simulink model "PowertrainElectrical"  (R2025a)
settings: Solver=VariableStepAuto  StartTime=0.0  StopTime=60  RelTol=1e-3
undefined symbols (not defined in the file): canChannel, Data, ID, Ts_PID, w_max
libraries: canlib x3, ESys x3, simulink x1, slpidlib x1
settings Model: DataDictionary=System.sldd  Creator=tecnicomcbti  LastModifiedBy=tecnicomcbti

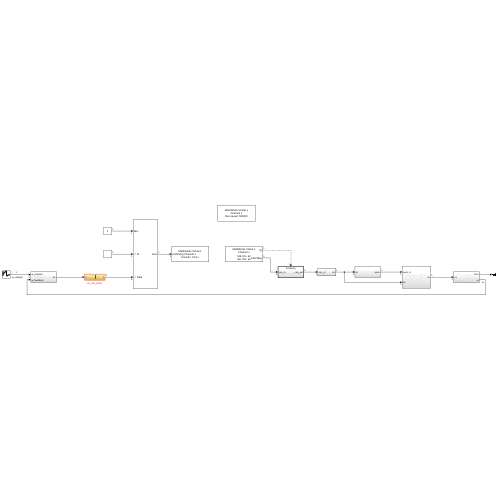
[thumbnail: Simulink's stored preview of the top-level diagram]
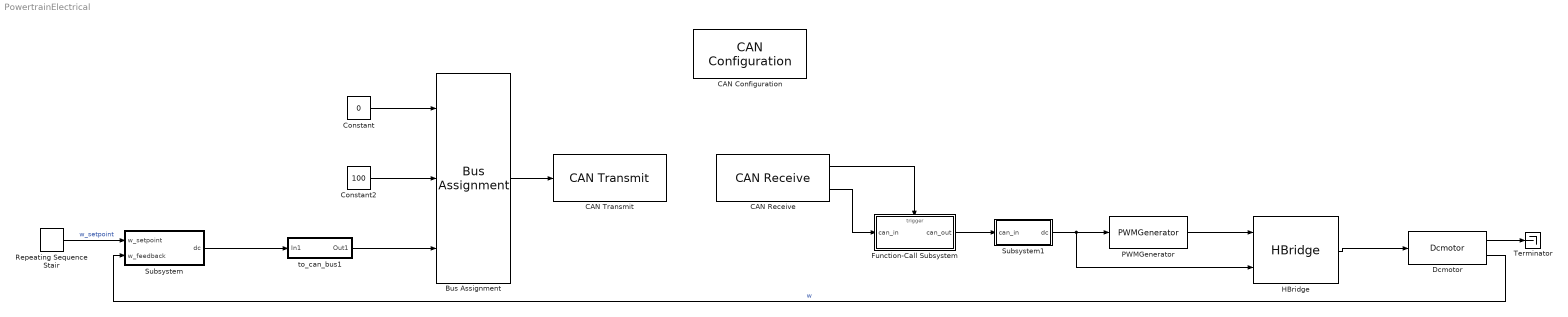
== system PowertrainElectrical ==
  Bus Assignment : BusAssignment  AssignedSignals=ID,Data
  CAN Configuration : canlib/CAN Configuration  BlockHandle=224.0002  Device=MathWorks Virtual 1 (Channel 1)  DeviceMenu=MathWorks Virtual 1 (Channel 1)  ObjConstructor=canChannel('MathWorks', 'Virtual 1', 1)  BusSpeed=500000  EnableBitParameters=off  AckMode=Normal
  CAN Receive : canlib/CAN Receive  BlockHandle=225.0002  Device=MathWorks Virtual 1 (Channel 1)  DeviceMenu=MathWorks Virtual 1 (Channel 1)  ObjConstructor=canChannel('MathWorks', 'Virtual 1', 1)  EnableStandardIDsFilter=off  StdIDsCombo=Allow all  StandardIDs=0  EnableExtendedIDsFilter=off  ExtIDsCombo=Allow all  ExtendedIDs=0  SampleTime=10e-3  MsgsPerTimestep=1  InternalFilterUpdateStatus=on  BusOutput=on
  CAN Transmit : canlib/CAN Transmit  BlockHandle=228.0001  Device=MathWorks Virtual 1 (Channel 1)  DeviceMenu=MathWorks Virtual 1 (Channel 1)  ObjConstructor=canChannel('MathWorks', 'Virtual 1', 1)  EnableEventTransmit=off  EnablePeriodicTransmit=on  MessagePeriod=10e-3
  Constant : Constant  Value=0  OutDataTypeStr=Bus: CAN_MESSAGE_BUS
  Constant2 : Constant  Value=100  OutDataTypeStr=uint32
  Dcmotor : ESys/Dcmotor  SystemSampleTime=-1  VariantActivationTime=update diagram  EmptyChoice=off  PassThrough=off  PassThroughVariantControl=(default)  EmptyChoiceVariantControl=(default)  AllowFlexibleInterface=on  Latency=0  AutoFrameSizeCalculation=off
  Function-Call Subsystem : Subsystem  TreatAsAtomicUnit=on
  HBridge : ESys/HBridge  SystemSampleTime=-1  VariantActivationTime=update diagram  EmptyChoice=off  PassThrough=off  PassThroughVariantControl=(default)  EmptyChoiceVariantControl=(default)  AllowFlexibleInterface=on  Latency=0  AutoFrameSizeCalculation=off
  PWMGenerator : ESys/PWMGenerator  SystemSampleTime=-1  VariantActivationTime=update diagram  EmptyChoice=off  PassThrough=off  PassThroughVariantControl=(default)  EmptyChoiceVariantControl=(default)  AllowFlexibleInterface=on  Latency=0  AutoFrameSizeCalculation=off
  Repeating Sequence Stair : simulink/Sources/Repeating Sequence Stair  OutValues=[300 400 500 150 200 250].'  tsamp=10  OutMin=[]  OutMax=[]  OutDataTypeStr=double  OutputDataTypeScalingMode=double  OutDataType=fixdt(0,8)  ConRadixGroup=Best Precision: Vector-wise  OutScaling=2^-12
  Subsystem : Subsystem
  Subsystem1 : Subsystem
  Terminator : Terminator
  to_can_bus1 : Subsystem
  wires:
  CAN Receive/2 -> Function-Call Subsystem/1(can_in)
  Function-Call Subsystem/1(can_out) -> Subsystem1/1(can_in)
  Bus Assignment/1 -> CAN Transmit/1
  Constant2/1 -> Bus Assignment/2
  CAN Receive/1 -> Function-Call Subsystem/Trigger
  Repeating Sequence Stair/1 -> Subsystem/1(w_setpoint)  "w_setpoint"
  Subsystem/1(dc) -> to_can_bus1/1(In1)
  Subsystem1/1(dc) -> HBridge/2, PWMGenerator/1
  PWMGenerator/1 -> HBridge/1
  HBridge/1 -> Dcmotor/1
  Dcmotor/2 -> Subsystem/2(w_feedback)  "w"
  Dcmotor/1 -> Terminator/1
  Constant/1 -> Bus Assignment/1
  to_can_bus1/1(Out1) -> Bus Assignment/3

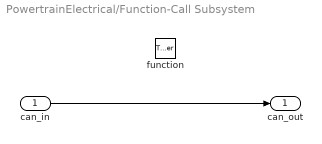
== system PowertrainElectrical/Function-Call Subsystem ==
  can_in : Inport
  function : TriggerPort  TriggerType=function-call  VariantControl=(inherit)
  can_out : Outport
  wires:
  can_in/1 -> can_out/1

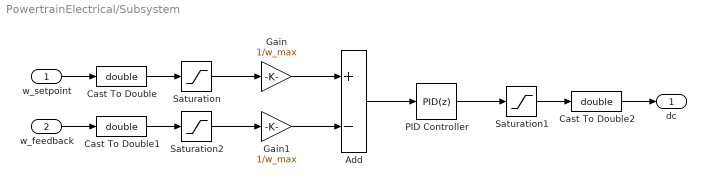
== system PowertrainElectrical/Subsystem ==
  w_setpoint : Inport
  w_feedback : Inport  Port=2
  Add : Sum  Inputs=+-
  Cast To Double : DataTypeConversion  OutDataTypeStr=double  SaturateOnIntegerOverflow=off  RndMeth=Floor
  Cast To Double1 : DataTypeConversion  OutDataTypeStr=double  SaturateOnIntegerOverflow=off  RndMeth=Floor
  Cast To Double2 : DataTypeConversion  OutDataTypeStr=double  SaturateOnIntegerOverflow=off  RndMeth=Floor
  Gain : Gain  Gain=1/w_max
  Gain1 : Gain  Gain=1/w_max
  PID Controller : slpidlib/PID Controller  Controller=PID  Form=Parallel  TimeDomain=Discrete-time  UseExternalTs=off  SampleTime=Ts_PID  IntegratorMethod=Forward Euler  FilterMethod=Forward Euler  ControllerParametersSource=internal  P=0.00488937991617763  I=0.977875983235526  UseKiTs=off  D=0  UseExternalDerivativeSource=off  N=100  UseFilter=on  TunerSelectOption=Transfer Function Based (PID Tuner App)  InitialConditionSource=internal  InitialConditionForIntegrator=0  InitialConditionForFilter=0  DifferentiatorICPrevScaledInput=0  ExternalReset=none  TrackingMode=off  Kt=1  LimitOutput=off  SatLimitsSource=internal  UpperSaturationLimit=inf  LowerSaturationLimit=-inf  LinearizeAsGain=on  AntiWindupMode=none  Kb=1  LimitIntegrator=off  UpperIntegratorSaturationLimit=inf  LowerIntegratorSaturationLimit=-inf  POutMin=[]  POutMax=[]  IOutMin=[]  IOutMax=[]  DOutMin=[]  DOutMax=[]  NOutMin=[]  NOutMax=[]  SumOutMin=[]  SumOutMax=[]  SaturationOutMin=[]  SaturationOutMax=[]  PParamMin=[]  PParamMax=[]  IParamMin=[]  IParamMax=[]  DParamMin=[]  DParamMax=[]  NParamMin=[]  NParamMax=[]  KbParamMin=[]  KbParamMax=[]  KtParamMin=[]  KtParamMax=[]  KbOutMin=[]  KbOutMax=[]  KtOutMin=[]  KtOutMax=[]  IntegratorOutMin=[]  IntegratorOutMax=[]  FilterOutMin=[]  FilterOutMax=[]  SumI1OutMin=[]  SumI1OutMax=[]  SumI2OutMin=[]  SumI2OutMax=[]  SumI3OutMin=[]  SumI3OutMax=[]  SumI4OutMin=[]  SumI4OutMax=[]  SumDOutMin=[]  SumDOutMax=[]  DifferentiatorOutMin=[]  DifferentiatorOutMax=[]  FilterDiffOutCoefMin=[]  FilterDiffOutCoefMax=[]  ReciprocalOutMin=[]  ReciprocalOutMax=[]  SumDenOutMin=[]  SumDenOutMax=[]  SumNumOutMin=[]  SumNumOutMax=[]  DivideOutMin=[]  DivideOutMax=[]  UdiffTsProdOutMin=[]  UdiffTsProdOutMax=[]  NTsProdOutMin=[]  NTsProdOutMax=[]  UintegralTsProdOutMin=[]  UintegralTsProdOutMax=[]  UngainTsProdOutMin=[]  UngainTsProdOutMax=[]  ClampingZeroOutDataTypeStr=Inherit: Inherit via back propagation  ClampingZeroOutMin=[]  ClampingZeroOutMax=[]  FilterDenConstantOutDataTypeStr=Inherit: Inherit via back propagation  FilterDenConstantOutMin=[]  FilterDenConstantOutMax=[]  PCopyOutDataTypeStr=Inherit: Inherit via back propagation  PCopyOutMin=[]  PCopyOutMax=[]  NCopyOutDataTypeStr=Inherit: Inherit via back propagation  NCopyOutMin=[]  NCopyOutMax=[]  IntegratorContinuousStateAttributes=''  IntegratorStateMustResolveToSignalObject=off  IntegratorRTWStateStorageClass=Auto  FilterContinuousStateAttributes=''  FilterStateMustResolveToSignalObject=off  FilterRTWStateStorageClass=Auto  ParallelPVariant=InternalParameters  IdealPVariant=Disabled  IVariant=InternalParameters  DVariant=InternalParameters  IntegratorVariant=Discrete  SatVariant=Disabled  AWVariant=Passthrough  PCopyVariant=Disabled  TRVariant=Disabled  FdbkBlocksVariant=Forward  IdealPFdbkVariant=Disabled  SatFdbkVariant=Disabled  DerivativeFilterVariant=ForwardEulerFilter  NVariant=InternalParameters  NCopyVariant=Disabled  FilterICVariant=InternalICsFilter  IntegratorICVariant=InternalICs  ExternalResetVariant=Disabled  TRSumVariant=Passthrough  SumFdbkVariant=Disabled  SumVariant=Sum_PID  TsampFilterVariant=InternalTs  TsampNgainVariant=Passthrough  TsampIntegralVariant=Disabled_SignalSpec  ExternalSaturationOutDataTypeStr=Inherit: Same as second input  DerivativeSourceVariant=ErrorSignal  PreIntVariant=InternalPreInt
  Saturation : Saturate  UpperLimit=w_max  LowerLimit=0
  Saturation1 : Saturate  UpperLimit=1  LowerLimit=0
  Saturation2 : Saturate  UpperLimit=w_max  LowerLimit=0
  dc : Outport
  wires:
  Add/1 -> PID Controller/1
  Gain/1 -> Add/1
  Cast To Double1/1 -> Saturation2/1
  w_setpoint/1 -> Cast To Double/1
  PID Controller/1 -> Saturation1/1
  Cast To Double2/1 -> dc/1
  Saturation1/1 -> Cast To Double2/1
  Saturation/1 -> Gain/1
  Saturation2/1 -> Gain1/1
  w_feedback/1 -> Cast To Double1/1
  Gain1/1 -> Add/2
  Cast To Double/1 -> Saturation/1

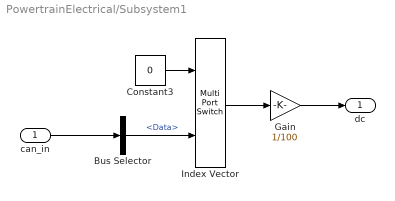
== system PowertrainElectrical/Subsystem1 ==
  can_in : Inport
  Bus Selector : BusSelector  OutputSignals=Data
  Constant3 : Constant  Value=0
  Gain : Gain  Gain=1/100
  Index Vector : MultiPortSwitch  DataPortOrder=Zero-based contiguous  Inputs=1  zeroidx=on  SaturateOnIntegerOverflow=off  InputSameDT=off
  dc : Outport
  wires:
  Gain/1 -> dc/1
  can_in/1 -> Bus Selector/1
  Constant3/1 -> Index Vector/1
  Index Vector/1 -> Gain/1
  Bus Selector/1 -> Index Vector/2  "<Data>"

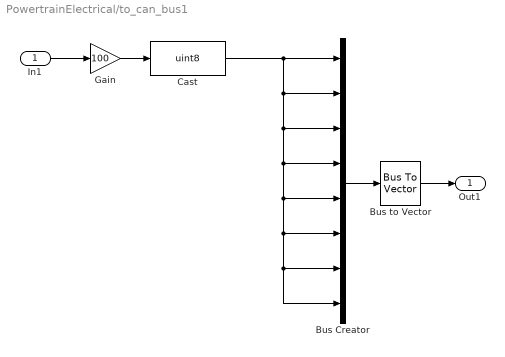
== system PowertrainElectrical/to_can_bus1 ==
  In1 : Inport
  Bus Creator : BusCreator  Inputs=8
  Bus to Vector : BusToVector
  Cast : DataTypeConversion  OutDataTypeStr=uint8  SaturateOnIntegerOverflow=off  RndMeth=Floor
  Gain : Gain  Gain=100
  Out1 : Outport
  wires:
  Bus to Vector/1 -> Out1/1
  Bus Creator/1 -> Bus to Vector/1
  Cast/1 -> Bus Creator/1, Bus Creator/2, Bus Creator/3, Bus Creator/4, Bus Creator/5, Bus Creator/6, Bus Creator/7, Bus Creator/8
  In1/1 -> Gain/1
  Gain/1 -> Cast/1
